simulink model "SOC_Regler"  (R2025b)
settings: Solver=VariableStepAuto  StartTime=0.0  StopTime=10.0  RelTol=1e-3
libraries: simulink x3
settings Model: DataDictionary=EScooter_Interfaces.sldd  Creator=jonas  LastModifiedBy=louis

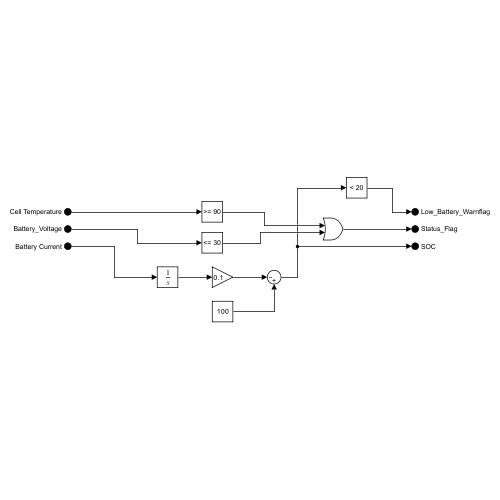
[thumbnail: Simulink's stored preview of the top-level diagram]
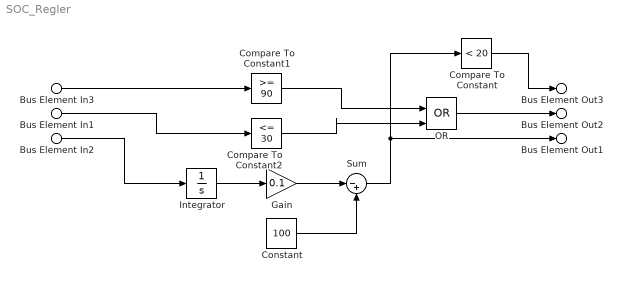
== system SOC_Regler ==
  Bus Element In3 : Inport  PortName=Cell Temperature
  Bus Element In1 : Inport  Port=2  PortName=Battery_Voltage
  Bus Element In2 : Inport  Port=3  PortName=Battery Current
  Compare To Constant : simulink/Logic and Bit Operations/Compare To Constant  relop=<  const=20  OutDataTypeStr=boolean
  Compare To Constant1 : simulink/Logic and Bit Operations/Compare To Constant  relop=>=  const=90  OutDataTypeStr=boolean
  Compare To Constant2 : simulink/Logic and Bit Operations/Compare To Constant  relop=<=  const=30  OutDataTypeStr=boolean
  Constant : Constant  Value=100
  Gain : Gain  Gain=0.1
  Integrator : Integrator
  OR : Logic  Operator=OR  IconShape=distinctive  AllPortsSameDT=off  OutDataTypeStr=boolean
  Sum : Sum  Inputs=|-+
  Bus Element Out3 : Outport  PortName=Low_Battery_Warnflag
  Bus Element Out2 : Outport  Port=2  PortName=Status_Flag
  Bus Element Out1 : Outport  Port=3  PortName=SOC
  wires:
  Bus Element In2/1 -> Integrator/1
  Integrator/1 -> Gain/1
  Gain/1 -> Sum/1
  Constant/1 -> Sum/2
  Compare To Constant/1 -> Bus Element Out3/1
  Sum/1 -> Bus Element Out1/1, Compare To Constant/1
  Bus Element In3/1 -> Compare To Constant1/1
  Bus Element In1/1 -> Compare To Constant2/1
  Compare To Constant1/1 -> OR/1
  Compare To Constant2/1 -> OR/2
  OR/1 -> Bus Element Out2/1
